simulink model "simulation_upgrade"  (R2024b)
settings: Solver=ode1be  StartTime=0.0  StopTime=10  FixedStep=0.001  RelTol=1e-3
model workspace (MAT data in the model file):
  AMP = 1
  FREQ = 1
  i_abc = 1
values from neighbouring files (symbols this model uses):
  v_WLTP = [0 0 0 0 0 0 0 0 0 0 0 0 ... (180001 elements, 1x180001)]    [v_WLTP.mat]
undefined symbols (not defined in the file or in its folder): A, a_sig, b_sig, C1, C2, C3, Cd, CG_z, downshift, Drive_wheel, Driveshaft, f_blend, f_OVD, fo, front_seat_dist, fs, g, Gearbox, i, i_sig, Inclination, Inertia, Jr2, K, m, M_curve_1, M_curve_2, m_driver, M_N_1, M_N_2, mi_c, mi_s, Mode, N_clutch, n_curve_1, n_curve_2, n_driver, n_max_1, n_max_2, n_shift, n_surfaces, Pl, Planetary, r_eq_clutch, r_geom, r_wheel, rho, Shaft, shift_time, sigma0, sigma1, sigma2, slope_angle, Stage1, Stage2, Stage3, upshift, v0, vel_wind, vs ... (+5)
libraries: simulink x29, slpidlib x3
(part 1 of 9)
settings Model: Creator=menda  LastModifiedBy=menda
settings SolverCC: ZeroCrossAlgorithm=Adaptive
settings DebuggingCC: AlgebraicLoopMsg=none  IgnoredZcDiagnostic=none

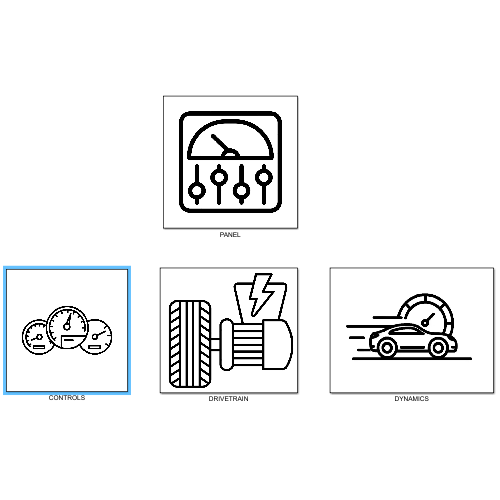
[thumbnail: Simulink's stored preview of the top-level diagram]
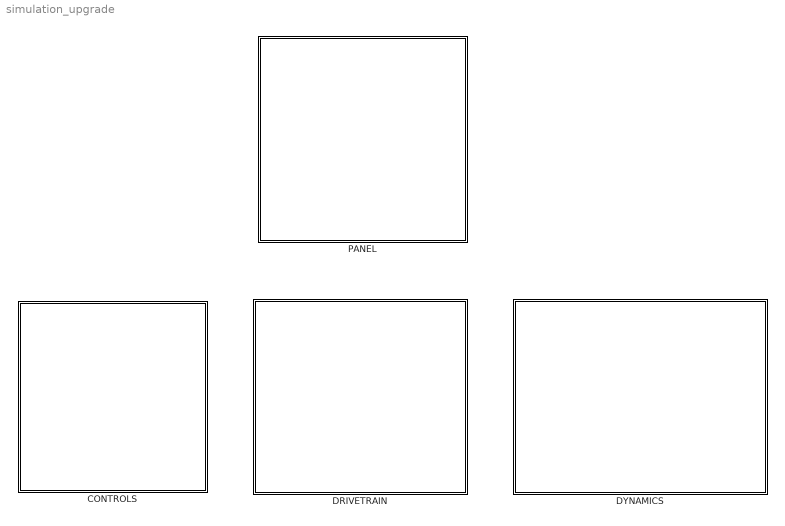
== system simulation_upgrade ==
  CONTROLS : Subsystem
      mask Display: image('images/controls.jpg');
  DRIVETRAIN : Subsystem
      mask Display: image('images/drivetrain_icon.png');
  DYNAMICS : Subsystem
      mask Display: image('images/Dynamics.png');
  PANEL : Subsystem
      mask Display: image('images/panel.jpg');

== system simulation_upgrade/CONTROLS ==
  Main Control Unit : Subsystem  Variant=on
      mask Display: image('images/MCU.jpg');
  Speed Profile : Subsystem
      mask Display: image('images/speedProfile.png');
  Speed control : Subsystem
      mask Display: image('images/speedControl.jpg');
  tag scope: Gear=global, M_MCU=global
  wires:
  Speed Profile/1(V/A) -> Speed control/2(v Target)  "v/a"
  Speed control/1(M) -> Main Control Unit/1(M_Driver)
  [Speed] -> Speed control/1(V fdbk)
  Main Control Unit/1(M_MCU) -> [M_MCU]  "Torque"
  Main Control Unit/2(Gear) -> [Gear]  "Gear"

== system simulation_upgrade/DRIVETRAIN ==
  Engine : Subsystem  Variant=on
      mask Display: image('images/engine.jpg');
  Transmission : Subsystem
      mask Display: image('images/transmission.jpg');
  Wheel Model : Subsystem
      mask Display: image('images/wheel_model.jpg');
  Zero : Constant  Value=0  OutDataTypeStr=Inherit: Inherit via back propagation
  tag scope: F_wheel=global, M_engine=global
  wires:
  Engine/1(M_engine) -> Transmission/1(M_engine), [M_engine]
  Wheel Model/1("  ") -> [F_wheel]  "F_wheels"
  [M_MCU] -> Engine/1(M_MCU)
  Zero/1 -> Wheel Model/3(M_break)
  Transmission/1(M_tra) -> Wheel Model/2(M_tra)
  [V_load] -> Wheel Model/1(Vload)

== system simulation_upgrade/DYNAMICS ==
  Aerodynamic Forces : Subsystem
      mask Display: image('images/aerodynamic.png');
  Inclination : Subsystem
      mask Display: image('images/slope.jpg');
  Load Transfer : Subsystem
      mask Display: image('images/Load_transfer.png');
  Rolling Resistance : Subsystem
      mask Display: image('images/rolling_resistance.png');
  Sum : Sum  Inputs=-+-
  Vehicle Dynamics : Subsystem
      mask Display: image('images/Dynamics.png');
  tag scope: Speed=global, V_load=global
  wires:
  Sum/1 -> Vehicle Dynamics/1(Ft)  "F_tractive"
  Rolling Resistance/1(F) -> Sum/2  "Fx"
  Inclination/1(F_G) -> Sum/3  "F_G"
  Aerodynamic Forces/1(Fa) -> Sum/1  "D_A"
  Vehicle Dynamics/1(v) -> [Speed]  "v"
  [Speed] -> Aerodynamic Forces/1(v_x), Rolling Resistance/1(v_x)
  Load Transfer/1(Fz) -> [V_load]
  Vehicle Dynamics/2(acc) -> Load Transfer/1(acc)
  Inclination/2(theta) -> Load Transfer/2(theta)
  [F_wheel] -> Rolling Resistance/2(Fw)
  [V_load] -> Rolling Resistance/3(Fz)

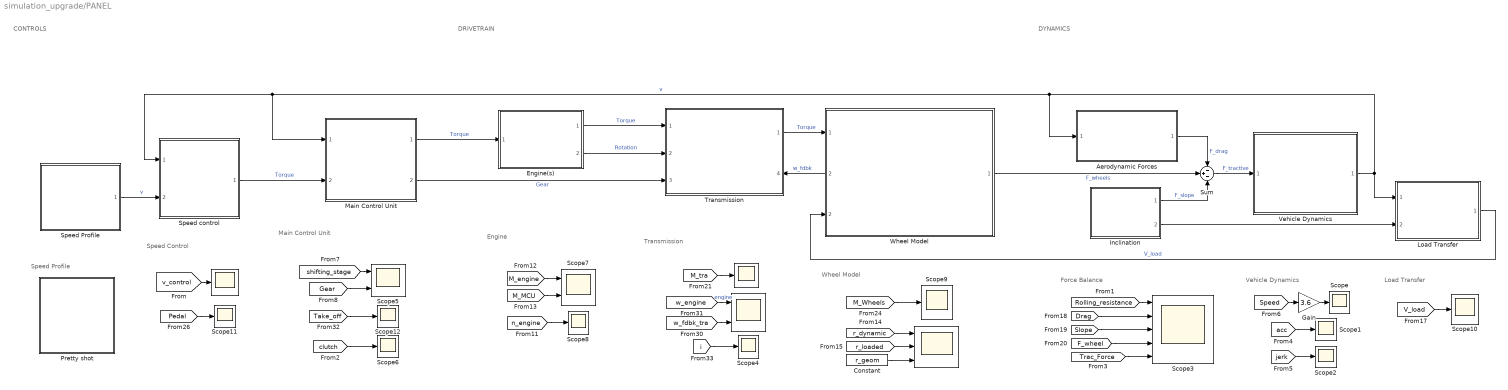
== system simulation_upgrade/PANEL ==
  note: Load Transfer
  note: Vehicle Dynamics
  note: Force Balance
  note: Speed Profile
  note: Transmission
  note: Main Control Unit
  note: Speed Control
  note: DYNAMICS
  note: CONTROLS
  note: DRIVETRAIN
  note: Engine
  note: Wheel Model
  " " : Scope
  "  " : Scope  NumInputPorts=3
  "        " : Scope  NumInputPorts=2
  "                " : Scope
  Aerodynamic Forces : Subsystem
      mask Display: image('images/aerodynamic.png');
  Constant : Constant  Value=r_geom
  Engine(s) : Subsystem
      mask Display: image('images/engine.jpg');
  Gain : Gain  Gain=3.6
  Inclination : Subsystem
      mask Display: image('images/slope.jpg');
  Load Transfer : Subsystem
      mask Display: image('images/Load_transfer.png');
  Main Control Unit : Subsystem
      mask Display: image('images/MCU.jpg');
  Pretty shot : Subsystem
  Scope{,1..2,4,6,8..12} (10 alike) : Scope
  Scope3 : Scope  NumInputPorts=5
  Scope5 : Scope  NumInputPorts=2
  Scope7 : Scope  NumInputPorts=2
  Speed Profile : Subsystem
      mask Display: image('images/speedProfile.png');
  Speed control : Subsystem
      mask Display: image('images/speedControl.jpg');
  Sum : Sum  Inputs=-+-
  Transmission : Subsystem
      settings: PortSchema="{\"entries\":[{\"content\":{\"sides\":[{\"content\":{\"connectorIds\":[\"In1\",\"In2\",\"In3\"]},\"type\":\"ConnectorPlacement.EquallySpacedRectSide\",\"uuid\":\"938dd209-6296-408a-9216-1c78db94ab7e\"},{\"content\":{\"connectorIds\":[\"Out1\",\"In4\"],\"side\":\"RIGHT\"},\"type\":\"ConnectorPlacement.EquallySpacedRectSide\",\"uuid\":\"09e50ecb-d14d-4cb9-a827-f943ac6e708a\"},{\"content\":{\"side\":\"TOP\"},\"type\":\"ConnectorPlacement.EquallySpacedRectSide\",\"uuid\":\"2d9a187e-939f-4518-982a-97ec647a77f4\"}]},\"type\":\"ConnectorPlacement.EquallySpacedConnector\",\"uuid\":\"677d1034-9393-4137-a143-928c8b2a4264\"}],\"packageUris\":[\"http://schema.mathworks.com/mf0/Connector/R2020b\"],\"version\":\"1.0\"}"
      mask Display: image('images/transmission.jpg');
  Vehicle Dynamics : Subsystem
      mask Display: image('images/Dynamics.png');
  Wheel Model : Subsystem
      settings: PortSchema="{\"entries\":[{\"content\":{\"sides\":[{\"content\":{\"connectorIds\":[\"In1\",\"Out2\",\"In2\"]},\"type\":\"ConnectorPlacement.EquallySpacedRectSide\",\"uuid\":\"938dd209-6296-408a-9216-1c78db94ab7e\"},{\"content\":{\"connectorIds\":[\"Out1\"],\"side\":\"RIGHT\"},\"type\":\"ConnectorPlacement.EquallySpacedRectSide\",\"uuid\":\"09e50ecb-d14d-4cb9-a827-f943ac6e708a\"},{\"content\":{\"side\":\"TOP\"},\"type\":\"ConnectorPlacement.EquallySpacedRectSide\",\"uuid\":\"2d9a187e-939f-4518-982a-97ec647a77f4\"}]},\"type\":\"ConnectorPlacement.EquallySpacedConnector\",\"uuid\":\"677d1034-9393-4137-a143-928c8b2a4264\"}],\"packageUris\":[\"http://schema.mathworks.com/mf0/Connector/R2020b\"],\"version\":\"1.0\"}"
      mask Display: image('images/wheel_model.jpg');
  wires:
  [v_control] -> "                "/1
  [Speed] -> Gain/1
  [acc] -> Scope1/1
  [Trac_Force] -> Scope3/5
  [jerk] -> Scope2/1
  [Gear] -> Scope5/2
  [shifting_stage] -> Scope5/1
  [M_engine] -> Scope7/1
  [M_MCU] -> Scope7/2
  [n_engine] -> Scope8/1
  Inclination/1(" ") -> Sum/3  "F_slope"
  Sum/1 -> Vehicle Dynamics/1(" ")  "F_tractive"
  Load Transfer/1("  ") -> Wheel Model/2("  ")  "V_load"
  Speed Profile/1(" ") -> Speed control/2("    ")  "v"
  Main Control Unit/1("    ") -> Engine(s)/1("  ")  "Torque"
  Aerodynamic Forces/1("  ") -> Sum/1  "F_drag"
  Vehicle Dynamics/1("  ") -> Aerodynamic Forces/1(" "), Speed control/1(" "), Main Control Unit/1(" "), Load Transfer/1(" ")  "v"
  Engine(s)/1("             ") -> Transmission/1(" ")  "Torque"
  Wheel Model/1("   ") -> Sum/2  "F_wheels"
  Transmission/1("  ") -> Wheel Model/1(" ")  "Torque"
  Speed control/1("        ") -> Main Control Unit/2("   ")  "Torque"
  Main Control Unit/2("  ") -> Transmission/3("    ")  "Gear"
  [r_dynamic] -> "  "/1
  [r_loaded] -> "  "/2
  Constant/1 -> "  "/3
  [V_load] -> Scope10/1
  [Drag] -> Scope3/2
  [Slope] -> Scope3/3
  [F_wheel] -> Scope3/4
  Inclination/2("   ") -> Load Transfer/2("      ")
  [M_tra] -> " "/1
  [M_Wheels] -> Scope9/1
  [Pedal] -> Scope11/1
  [w_fdbk_tra] -> "        "/2
  Gain/1 -> Scope/1
  [w_engine] -> "        "/1  "engine"
  [Take_off] -> Scope12/1
  [i] -> Scope4/1
  Wheel Model/2("    ") -> Transmission/4("   ")  "w_fdbk"
  Engine(s)/2("              ") -> Transmission/2("     ")  "Rotation"
  [Rolling_resistance] -> Scope3/1
  [clutch] -> Scope6/1

== system simulation_upgrade/CONTROLS/Main Control Unit ==
  note: 1) Add Subsystem or Model blocks as valid variant choices.
      | 2) You cannot connect blocks at this level. At simulation, connectivity is automatically
      | determined, based on the active variant and port name matching.
  M_Driver : Inport
  AMT_MCU : Subsystem  VariantControl=Gearbox == 2
  AT_MCU : Subsystem  VariantControl=Gearbox == 1
  CVT_MCU : Subsystem  VariantControl=Gearbox == 5
  DCT_MCU : Subsystem  VariantControl=Gearbox == 3
  TDT_MCU : Subsystem  VariantControl=Gearbox == 4
  M_MCU : Outport
  Gear : Outport  Port=2

== system simulation_upgrade/CONTROLS/Speed Profile ==
  0% Pedal : Step  Time=0  After=0  SampleTime=0
  AND : Logic  IconShape=distinctive  AllPortsSameDT=off  OutDataTypeStr=boolean
  Add3 : Sum
  Bus Creator : BusCreator  Inputs=2
  Compare To Constant2 : simulink/Logic and Bit Operations/Compare To Constant  relop=>=  const=2  OutDataTypeStr=boolean
  Compare To Constant3 : simulink/Logic and Bit Operations/Compare To Constant  relop=<  const=0.01  OutDataTypeStr=boolean
  Constant : Constant  Value=Mode
  Constant12 : Constant  Value=0.3
  Constant13 : Constant  Value=0
  Constant14 : Constant  Value=0
  Constant15 : Constant  Value=-0.6
  Digital Clock : DigitalClock  SampleTime=0.001
  Digital Clock1 : DigitalClock  SampleTime=0.01
  Gain : Gain  Gain=3.6
  Ramp1 : simulink/Sources/Ramp  slope=1  start=0  InitialOutput=0
  Ramp2 : simulink/Sources/Ramp  slope=-0.5  start=10  InitialOutput=0
  Saturation Dynamic : simulink/Discontinuities/Saturation Dynamic  OutMin=[]  OutMax=[]  OutDataTypeStr=Inherit: Same as second input  OutDataType=fixdt(1, 16)  OutScaling=2^-10  DoSatur=off
  Saturation Dynamic1 : simulink/Discontinuities/Saturation Dynamic  OutMin=[]  OutMax=[]  OutDataTypeStr=Inherit: Same as second input  OutDataType=fixdt(1, 16)  OutScaling=2^-10  DoSatur=off
  Scope25 : Scope
  Scope26 : Scope
  Setpoint Speed (Acceleration) : Step  Time=0  After=80  SampleTime=0
  Setpoint Speed (Acceleration)1 : Step  Time=10  After=-80  SampleTime=0
  Sum : Sum  Inputs=|++
  Switch : Switch  Criteria=u2 > Threshold  Threshold=1  SaturateOnIntegerOverflow=off  InputSameDT=off
  Switch2 : Switch  Criteria=u2 > Threshold  SaturateOnIntegerOverflow=off  InputSameDT=off
  WLTP Profile : Lookup_n-D  NumberOfTableDimensions=1  BreakpointsForDimension1=t  Table=v_WLTP  InternalRulePriority=Speed  RndMeth=Simplest
  V/A : Outport
  wires:
  Setpoint Speed (Acceleration)1/1 -> Sum/2
  Setpoint Speed (Acceleration)/1 -> Sum/1
  Digital Clock/1 -> WLTP Profile/1
  WLTP Profile/1 -> Switch/1
  Constant/1 -> Switch/2
  Sum/1 -> Switch/3
  Switch/1 -> Bus Creator/2  "v_target"
  Constant12/1 -> Saturation Dynamic1/1
  Digital Clock1/1 -> Compare To Constant2/1
  Constant14/1 -> Saturation Dynamic/1
  [Speed] -> Gain/1
  Saturation Dynamic/1 -> Add3/1
  Switch2/1 -> Scope26/1, Bus Creator/1  "pedal"
  Compare To Constant2/1 -> AND/1
  Ramp2/1 -> Saturation Dynamic/2
  AND/1 -> Switch2/2
  Saturation Dynamic1/1 -> Add3/2
  Constant13/1 -> Saturation Dynamic1/3
  Compare To Constant3/1 -> AND/2
  Gain/1 -> Compare To Constant3/1  "v_ist"
  Constant15/1 -> Saturation Dynamic/3
  Add3/1 -> Switch2/3, Scope25/1
  0% Pedal/1 -> Switch2/1  "Pedal Value Limited"
  Ramp1/1 -> Saturation Dynamic1/2
  Bus Creator/1 -> V/A/1

== system simulation_upgrade/CONTROLS/Speed control ==
  V fdbk : Inport
  v Target : Inport  Port=2
  Add : Sum  Inputs=+-
  Bus Creator : BusCreator  Inputs=3
  Bus Selector : BusSelector  OutputSignals=pedal,v_target
  Constant : Constant  Value=Mode
  Constant1 : Constant  Value=Gearbox
  Gain : Gain  Gain=3.6
  Gain1 : Gain  Gain=M_N_1
  Gain2 : Gain  Gain=M_N_2
  Pedal Value Limiter : Saturate  UpperLimit=1  LowerLimit=-1
  Speed Control : slpidlib/PID Controller  Controller=PID  Form=Parallel  TimeDomain=Continuous-time  UseExternalTs=off  SampleTime=-1  IntegratorMethod=Forward Euler  FilterMethod=Forward Euler  ControllerParametersSource=internal  P=0.8  I=0.001  UseKiTs=off  D=0  UseExternalDerivativeSource=off  N=100  UseFilter=on  TunerSelectOption=Transfer Function Based (PID Tuner App)  InitialConditionSource=internal  InitialConditionForIntegrator=0  InitialConditionForFilter=0  DifferentiatorICPrevScaledInput=0  ExternalReset=none  TrackingMode=off  Kt=1  LimitOutput=off  SatLimitsSource=internal  UpperSaturationLimit=inf  LowerSaturationLimit=-inf  LinearizeAsGain=on  AntiWindupMode=none  Kb=1  LimitIntegrator=off  UpperIntegratorSaturationLimit=inf  LowerIntegratorSaturationLimit=-inf  POutMin=[]  POutMax=[]  IOutMin=[]  IOutMax=[]  DOutMin=[]  DOutMax=[]  NOutMin=[]  NOutMax=[]  SumOutMin=[]  SumOutMax=[]  SaturationOutMin=[]  SaturationOutMax=[]  PParamMin=[]  PParamMax=[]  IParamMin=[]  IParamMax=[]  DParamMin=[]  DParamMax=[]  NParamMin=[]  NParamMax=[]  KbParamMin=[]  KbParamMax=[]  KtParamMin=[]  KtParamMax=[]  KbOutMin=[]  KbOutMax=[]  KtOutMin=[]  KtOutMax=[]  IntegratorOutMin=[]  IntegratorOutMax=[]  FilterOutMin=[]  FilterOutMax=[]  SumI1OutMin=[]  SumI1OutMax=[]  SumI2OutMin=[]  SumI2OutMax=[]  SumI3OutMin=[]  SumI3OutMax=[]  SumI4OutMin=[]  SumI4OutMax=[]  SumDOutMin=[]  SumDOutMax=[]  DifferentiatorOutMin=[]  DifferentiatorOutMax=[]  FilterDiffOutCoefMin=[]  FilterDiffOutCoefMax=[]  ReciprocalOutMin=[]  ReciprocalOutMax=[]  SumDenOutMin=[]  SumDenOutMax=[]  SumNumOutMin=[]  SumNumOutMax=[]  DivideOutMin=[]  DivideOutMax=[]  UdiffTsProdOutMin=[]  UdiffTsProdOutMax=[]  NTsProdOutMin=[]  NTsProdOutMax=[]  UintegralTsProdOutMin=[]  UintegralTsProdOutMax=[]  UngainTsProdOutMin=[]  UngainTsProdOutMax=[]  ClampingZeroOutDataTypeStr=Inherit: Inherit via back propagation  ClampingZeroOutMin=[]  ClampingZeroOutMax=[]  FilterDenConstantOutDataTypeStr=Inherit: Inherit via back propagation  FilterDenConstantOutMin=[]  FilterDenConstantOutMax=[]  PCopyOutDataTypeStr=Inherit: Inherit via back propagation  PCopyOutMin=[]  PCopyOutMax=[]  NCopyOutDataTypeStr=Inherit: Inherit via back propagation  NCopyOutMin=[]  NCopyOutMax=[]  IntegratorContinuousStateAttributes=''  IntegratorStateMustResolveToSignalObject=off  IntegratorRTWStateStorageClass=Auto  FilterContinuousStateAttributes=''  FilterStateMustResolveToSignalObject=off  FilterRTWStateStorageClass=Auto  ParallelPVariant=InternalParameters  IdealPVariant=Disabled  IVariant=InternalParameters  DVariant=InternalParameters  IntegratorVariant=Continuous  SatVariant=Disabled  AWVariant=Passthrough  PCopyVariant=Disabled  TRVariant=Disabled  FdbkBlocksVariant=Forward  IdealPFdbkVariant=Disabled  SatFdbkVariant=Disabled  DerivativeFilterVariant=ContFilter  NVariant=InternalParameters  NCopyVariant=Disabled  FilterICVariant=InternalICsFilter  IntegratorICVariant=InternalICs  ExternalResetVariant=Disabled  TRSumVariant=Passthrough  SumFdbkVariant=Disabled  SumVariant=Sum_PID  TsampFilterVariant=InternalTs  TsampNgainVariant=Passthrough  TsampIntegralVariant=Disabled_SignalSpec  ExternalSaturationOutDataTypeStr=Inherit: Same as second input  DerivativeSourceVariant=ErrorSignal  PreIntVariant=InternalPreInt
  Sum : Sum  Inputs=|++
  Switch : Switch  Criteria=u2 > Threshold  Threshold=2  SaturateOnIntegerOverflow=off  InputSameDT=off
  Switch1 : Switch  Criteria=u2 > Threshold  Threshold=3  SaturateOnIntegerOverflow=off  InputSameDT=off
  Transfer Fcn : TransferFcn  Denominator=[0.008 1]
  M : Outport
  tag scope: Pedal=global, v_control=global, v_error=global, v_fdbk=global, v_target=global
  wires:
  Add/1 -> Speed Control/1, [v_error]  "v_error"
  Speed Control/1 -> Pedal Value Limiter/1
  Switch1/1 -> M/1  "Setpoint Torque"
  V fdbk/1 -> Gain/1
  Gain/1 -> [v_fdbk], Add/2  "v_fdbk"
  Transfer Fcn/1 -> Gain1/1, Gain2/1, [Pedal]  "Pedal_value"
  Pedal Value Limiter/1 -> Switch/3
  Constant/1 -> Switch/2
  v Target/1 -> Bus Selector/1
  Bus Selector/1 -> Switch/1  "<pedal>"
  Gain1/1 -> Switch1/3, Sum/2
  Sum/1 -> Switch1/1
  Gain2/1 -> Sum/1
  Constant1/1 -> Switch1/2
  Switch/1 -> Transfer Fcn/1
  [v_target] -> Bus Creator/3  "v_target"
  [v_fdbk] -> Bus Creator/1  "v_fdbk"
  [v_error] -> Bus Creator/2  "v_error"
  Bus Creator/1 -> [v_control]
  Bus Selector/2 -> Add/1, [v_target]  "<v_target>"

== system simulation_upgrade/DRIVETRAIN/Engine ==
  note: 1) Add Subsystem or Model blocks as valid variant choices.
      | 2) You cannot connect blocks at this level. At simulation, connectivity is automatically
      | determined, based on the active variant and port name matching.
  M_MCU : Inport
  AMT_Engine : Subsystem  VariantControl=Gearbox == 2
  AT_Engine : Subsystem  VariantControl=Gearbox == 1
  DCT_Engine : Subsystem  VariantControl=Gearbox == 3
  TDT_Engine : Subsystem  VariantControl=Gearbox == 4
  e-CVT_Engine : Subsystem  VariantControl=Gearbox == 5
  M_engine : Outport

== system simulation_upgrade/DRIVETRAIN/Transmission ==
  M_engine : Inport
  Differential and Driveshafts : Subsystem
      mask Display: image('images/transmission.jpg');
  Gearbox : Subsystem  Variant=on
      mask Display: image('images/branco.png');
  eff_GB : Gain  Gain=0.97
  M_tra : Outport
  wires:
  M_engine/1 -> Gearbox/1(M_engine)
  Gearbox/1(M_Diff) -> eff_GB/1
  eff_GB/1 -> Differential and Driveshafts/1(M_Diff)
  Differential and Driveshafts/1(M_tra) -> M_tra/1

== system simulation_upgrade/DRIVETRAIN/Wheel Model ==
  Vload : Inport
  M_tra : Inport  Port=2
  M_break : Inport  Port=3
  Bus Creator : BusCreator  Inputs=2
  Bus Creator1 : BusCreator  Inputs=2
  Bus Creator2 : BusCreator  Inputs=2
  Bus Selector : BusSelector  OutputSignals=Rear_Vload,Front_Vload
  Constant5 : Constant  Value=Drive_wheel
  Divide2 : Product  Inputs=/*
  Front Wheels : Subsystem
      mask Display: image('images/branco.png');
  Integrator : Integrator
  Multiport Switch : MultiPortSwitch  DataPortOrder=Zero-based contiguous  zeroidx=on  SaturateOnIntegerOverflow=off  InputSameDT=off
  Rear Wheels : Subsystem
      mask Display: image('images/branco.png');
  Sum : Sum  Inputs=+|+
  "  " : Outport
  tag scope: M_Wheels=global, r_dynamic=global, r_loaded=global, w_fdbk_tire=global
  wires:
  Sum/1 -> "  "/1
  Vload/1 -> Bus Selector/1
  Bus Selector/1 -> Rear Wheels/3(Vload)  "<Rear_Vload>"
  Bus Selector/2 -> Front Wheels/1(Vload)  "<Front_Vload>"
  Rear Wheels/1(F_rear_wheels) -> Sum/1  "F_rear"
  Front Wheels/1(F_front_wheels) -> Sum/2  "F_front"
  M_tra/1 -> Rear Wheels/1(M_tra), Front Wheels/2(M_tra)
  M_break/1 -> Front Wheels/3(M_break), Rear Wheels/2(M_break)
  [acc] -> Divide2/2
  Multiport Switch/1 -> Divide2/1
  Integrator/1 -> [w_fdbk_tire]  "w_fdbk_tire"
  Constant5/1 -> Multiport Switch/1
  [r_dyn_rear] -> Bus Creator/2, Multiport Switch/4, Multiport Switch/2
  [r_dyn_front] -> Multiport Switch/3, Bus Creator/1
  Bus Creator/1 -> [r_dynamic]
  Bus Creator1/1 -> [r_loaded]
  [r_loaded_front] -> Bus Creator1/2
  [r_loaded_rear] -> Bus Creator1/1
  Divide2/1 -> Integrator/1
  [M_front_wheels] -> Bus Creator2/1
  [M_rear_wheels] -> Bus Creator2/2
  Bus Creator2/1 -> [M_Wheels]

== system simulation_upgrade/DYNAMICS/Aerodynamic Forces ==
  v_x : Inport
  Add : Sum  Inputs=+-
  Constant : Constant  Value=rho*A*0.5*Cd
  Constant1 : Constant  Value=vel_wind
  Math Function : Math  Operator=square  SignedPower=on
  Product : Product  RndMeth=Zero
  Product2 : Product  RndMeth=Zero
  Sign : Signum
  Fa : Outport  VectorParamsAs1DForOutWhenUnconnected=off
  tag scope: Drag=global
  wires:
  Add/1 -> Math Function/1
  Math Function/1 -> Product/2
  Sign/1 -> Product/1
  Constant/1 -> Product2/2
  Product2/1 -> [Drag], Fa/1  "Drag"
  Constant1/1 -> Add/2
  v_x/1 -> Add/1, Sign/1
  Product/1 -> Product2/1

== system simulation_upgrade/DYNAMICS/Inclination ==
  Constant : Constant  Value=slope_angle
  Constant1 : Constant  Value=Inclination
  Constant8 : Constant  Value=m+n_driver*m_driver
  Constant9 : Constant  Value=g
  Digital Clock : DigitalClock  Commented=on  SampleTime=0.01
  Product : Product  Inputs=3  RndMeth=Zero
  Slope Profile : Lookup_n-D  Commented=on  NumberOfTableDimensions=1  BreakpointsForDimension1=t  Table=i_sig  InternalRulePriority=Speed  RndMeth=Simplest
  Switch : Switch  Criteria=u2 > Threshold  SaturateOnIntegerOverflow=off  InputSameDT=off
  Trigonometric Function : Trigonometry
  F_G : Outport  VectorParamsAs1DForOutWhenUnconnected=off
  theta : Outport  Port=2  VectorParamsAs1DForOutWhenUnconnected=off
  tag scope: Slope=global
  wires:
  Product/1 -> F_G/1, [Slope]  "Slope"
  Constant9/1 -> Product/3
  Switch/1 -> theta/1, Trigonometric Function/1
  Trigonometric Function/1 -> Product/1
  Constant8/1 -> Product/2
  Constant/1 -> Switch/3
  Constant1/1 -> Switch/2
  Digital Clock/1 -> Slope Profile/1
  Slope Profile/1 -> Switch/1

== system simulation_upgrade/DYNAMICS/Load Transfer ==
  acc : Inport
  theta : Inport  Port=2
  Bus Creator : BusCreator  Inputs=2
  Constant : Constant  Value=g*WB_rear_dist
  Constant1 : Constant  Value=n_driver*m_driver*g*front_seat_dist
  Constant2 : Constant  Value=g*(1-WB_rear_dist)
  Constant3 : Constant  Value=n_driver*m_driver*g*(1-front_seat_dist)
  Cos : Trigonometry  Operator=cos
  Delay3 : Delay  DelayLength=1  InputProcessing=Columns as channels (frame based)
  Gain1 : Gain  Gain=CG_z/WB
  Product{,1..5} (6 alike) : Product
  Sum : Sum  Inputs=|++
  Sum1 : Sum  Inputs=-+|
  Sum2 : Sum  Inputs=++|
  Sum3 : Sum  Inputs=++|
  Fz : Outport
  tag scope: Vload_front=global, Vload_rear=global
  wires:
  Sum/1 -> Product/1
  Gain1/1 -> Sum/2, Sum1/1
  Sum1/1 -> Product1/2
  Sum3/1 -> Bus Creator/2, [Vload_front]  "Front_Vload"
  Sum2/1 -> Bus Creator/1, [Vload_rear]  "Rear_Vload"
  [m_eff] -> Product/2, Product1/1
  Constant/1 -> Product2/2
  Constant2/1 -> Product3/1
  Bus Creator/1 -> Fz/1
  acc/1 -> Delay3/1
  Delay3/1 -> Gain1/1
  Product/1 -> Sum2/1
  Product1/1 -> Sum3/1
  Constant1/1 -> Product4/1
  Constant3/1 -> Product5/2
  Product2/1 -> Sum/1
  Product3/1 -> Sum1/2
  theta/1 -> Cos/1
  Cos/1 -> Product4/2, Product2/1, Product3/2, Product5/1
  Product4/1 -> Sum2/2
  Product5/1 -> Sum3/2

== system simulation_upgrade/DYNAMICS/Rolling Resistance ==
  v_x : Inport
  Fw : Inport  Port=2
  Fz : Inport  Port=3
  Abs : Abs  SaturateOnIntegerOverflow=off
  Abs2 : Abs  SaturateOnIntegerOverflow=off
  Bus Selector : BusSelector  OutputSignals=Rear_Vload,Front_Vload
  Constant : Constant  Value=2.5
  Constant1 : Constant  Value=fo
  Delay : Delay  DelayLength=1  InputProcessing=Columns as channels (frame based)
  Gain : Gain  Gain=1/44.7
  Gain1 : Gain  Gain=3.24*fs
  Gain2 : Gain  Gain=-1
  Power : Math  Operator=pow
  Product : Product
  Saturation Dynamic : simulink/Discontinuities/Saturation Dynamic  OutMin=[]  OutMax=[]  OutDataTypeStr=Inherit: Same as second input  OutDataType=fixdt(1, 16)  OutScaling=2^-10  DoSatur=off
  Scope : Scope
  Step : Step  Time=0  After=0  SampleTime=0
  Sum : Sum  Inputs=|++
  Sum1 : Sum  Inputs=+-|
  Sum2 : Sum  Inputs=+|+
  Switch : Switch  SaturateOnIntegerOverflow=off  InputSameDT=off
  F : Outport
  tag scope: Rolling_resistance=global
  wires:
  Gain/1 -> Power/1
  Constant/1 -> Power/2
  Power/1 -> Gain1/1
  Gain1/1 -> Sum/1
  Constant1/1 -> Sum/2
  Sum/1 -> Scope/1, Product/2  "f_roll"
  Fz/1 -> Bus Selector/1
  Product/1 -> Switch/1
  Saturation Dynamic/1 -> Sum1/2, [Rolling_resistance]  "rolling_resistance"
  Fw/1 -> Sum1/1, Abs/1
  v_x/1 -> Delay/1
  Abs2/1 -> Switch/2
  Sum1/1 -> F/1
  Bus Selector/1 -> Sum2/1  "<Rear_Vload>"
  Sum2/1 -> Product/1
  Bus Selector/2 -> Sum2/2  "<Front_Vload>"
  Delay/1 -> Gain/1, Abs2/1
  Switch/1 -> Saturation Dynamic/2
  Gain2/1 -> Saturation Dynamic/3
  Step/1 -> Switch/3
  Abs/1 -> Gain2/1, Saturation Dynamic/1

== system simulation_upgrade/DYNAMICS/Vehicle Dynamics ==
  Ft : Inport
  Constant2 : Constant  Value=v0
  Derivative : Derivative
  Divide : Product  Inputs=*/
  Effective mass : Subsystem
  Integrator1 : Integrator  InitialConditionSource=external
  Saturation : Saturate  UpperLimit=3*m*g/2  LowerLimit=-3*m*g/2
  Scope : Scope  NumInputPorts=3
  Speed Saturation1 : Saturate  UpperLimit=2*pi*r_geom*n_max_1/(60*i.min)  LowerLimit=0
  v : Outport
  acc : Outport  Port=2
  tag scope: Trac_Force=global, acc=global, jerk=global
  wires:
  Ft/1 -> Saturation/1, Scope/1, [Trac_Force]  "F_tractive"
  Integrator1/1 -> Speed Saturation1/1  "v_x"
  Derivative/1 -> [jerk]
  Effective mass/1(m_eff) -> Divide/2
  Saturation/1 -> Divide/1, Scope/2
  Divide/1 -> Integrator1/1, Derivative/1, acc/1, Scope/3, [acc]  "acc"
  Constant2/1 -> Integrator1/2
  Speed Saturation1/1 -> v/1

== system simulation_upgrade/PANEL/Aerodynamic Forces ==
  " " : Inport
  "  " : Outport
  wires:
  " "/1 -> "  "/1

== system simulation_upgrade/PANEL/Engine(s) ==
  "  " : Inport
  "             " : Outport
  "              " : Outport  Port=2
  wires:
  "  "/1 -> "             "/1

== system simulation_upgrade/PANEL/Inclination ==
  Constant : Constant
  " " : Outport
  "   " : Outport  Port=2
  wires:
  Constant/1 -> "   "/1, " "/1

== system simulation_upgrade/PANEL/Load Transfer ==
  " " : Inport
  "      " : Inport  Port=2
  Terminator : Terminator
  "  " : Outport
  wires:
  " "/1 -> "  "/1
  "      "/1 -> Terminator/1

== system simulation_upgrade/PANEL/Main Control Unit ==
  " " : Inport
  "   " : Inport  Port=2
  Chart : Stateflow chart  Commented=on  TreatAsAtomicUnit=on
  "    " : Outport
  "  " : Outport  Port=2
  wires:
  " "/1 -> Chart/1(" ")
  "   "/1 -> Chart/2("   ")
  Chart/2("    ") -> "    "/1
  Chart/1("  ") -> "  "/1

== system simulation_upgrade/PANEL/Pretty shot ==
  "Aerodynamic Forces " : Subsystem
      mask Display: image('images/aerodynamic.png');
  "Engine(s) " : Subsystem
      settings: PortSchema="{\"entries\":[{\"content\":{\"sides\":[{\"content\":{},\"type\":\"ConnectorPlacement.EquallySpacedRectSide\",\"uuid\":\"ac5fb7f4-8dc2-4c60-98c0-b32a7c0962c0\"},{\"content\":{\"connectorIds\":[\"Out1\",\"Out2\"],\"side\":\"RIGHT\"},\"type\":\"ConnectorPlacement.EquallySpacedRectSide\",\"uuid\":\"b7133a62-cb88-4836-b384-7b1ee67f5a46\"},{\"content\":{\"connectorIds\":[\"In1\"],\"side\":\"TOP\"},\"type\":\"ConnectorPlacement.EquallySpacedRectSide\",\"uuid\":\"f8e13883-115b-42d7-970b-6e45a84dda6f\"},{\"content\":{\"side\":\"BOTTOM\"},\"type\":\"ConnectorPlacement.EquallySpacedRectSide\",\"uuid\":\"500f1a98-e247-4b4c-a18f-57d00a98d574\"}]},\"type\":\"ConnectorPlacement.EquallySpacedConnector\",\"uuid\":\"d392102a-fa12-401e-96eb-94eaccf256c5\"}],\"packageUris\":[\"http://schema.mathworks.com/mf0/Connector/R2020b\"],\"version\":\"1.0\"}"
      mask Display: image('images/engine2.jpg');
  "Inclination " : Subsystem
      mask Display: image('images/slope.jpg');
  "Load Transfer " : Subsystem
      settings: PortSchema="{\"entries\":[{\"content\":{\"sides\":[{\"content\":{\"connectorIds\":[\"In1\"]},\"type\":\"ConnectorPlacement.EquallySpacedRectSide\",\"uuid\":\"26581e23-f4af-4a6b-94dc-24984d7cf9dd\"},{\"content\":{\"connectorIds\":[\"Out1\",\"In2\"],\"side\":\"RIGHT\"},\"type\":\"ConnectorPlacement.EquallySpacedRectSide\",\"uuid\":\"dc974c34-bd2c-4374-a001-b5c53f67a3d1\"},{\"content\":{\"side\":\"TOP\"},\"type\":\"ConnectorPlacement.EquallySpacedRectSide\",\"uuid\":\"199156e0-9732-4241-ab5b-4e4dfddfabae\"}]},\"type\":\"ConnectorPlacement.EquallySpacedConnector\",\"uuid\":\"d2a32550-3940-404c-bc97-4724ab74b5d6\"}],\"packageUris\":[\"http://schema.mathworks.com/mf0/Connector/R2020b\"],\"version\":\"1.0\"}"
      mask Display: image('images/Load_transfer.png');
  "Main Control Unit " : Subsystem
      settings: PortSchema="{\"entries\":[{\"content\":{\"sides\":[{\"content\":{\"connectorIds\":[\"In1\",\"In2\"]},\"type\":\"ConnectorPlacement.EquallySpacedRectSide\",\"uuid\":\"b8fd4e6d-8e53-4c18-9f6d-747eb079d798\"},{\"content\":{\"connectorIds\":[\"Out1\"],\"side\":\"RIGHT\"},\"type\":\"ConnectorPlacement.EquallySpacedRectSide\",\"uuid\":\"2557e908-cd18-4a3e-b3a6-cb286cbd4d67\"},{\"content\":{\"side\":\"TOP\"},\"type\":\"ConnectorPlacement.EquallySpacedRectSide\",\"uuid\":\"b9022aa8-32dd-4520-9d7b-0035f068fa03\"},{\"content\":{\"connectorIds\":[\"Out2\"],\"side\":\"BOTTOM\"},\"type\":\"ConnectorPlacement.EquallySpacedRectSide\",\"uuid\":\"03495357-ab9a-4889-8bdc-80670051615f\"}]},\"type\":\"ConnectorPlacement.EquallySpacedConnector\",\"uuid\":\"266d5008-05ee-4fe5-82db-1148b4f01b90\"}],\"packageUris\":[\"http://schema.mathworks.com/mf0/Connector/R2020b\"],\"version\":\"1.0\"}"
      mask Display: image('images/MCU.jpg');
  "Speed Profile " : Subsystem
      settings: PortSchema="{\"entries\":[{\"content\":{\"sides\":[{\"content\":{},\"type\":\"ConnectorPlacement.EquallySpacedRectSide\",\"uuid\":\"ecf4b2d3-f448-439a-be96-5b35a4fd23fb\"},{\"content\":{\"side\":\"RIGHT\"},\"type\":\"ConnectorPlacement.EquallySpacedRectSide\",\"uuid\":\"9f661ef6-dada-4229-be93-12e76a82dfa4\"},{\"content\":{\"side\":\"TOP\"},\"type\":\"ConnectorPlacement.EquallySpacedRectSide\",\"uuid\":\"ac4e96df-6f30-4a9f-b005-38b2f14b4e0b\"},{\"content\":{\"connectorIds\":[\"Out1\"],\"side\":\"BOTTOM\"},\"type\":\"ConnectorPlacement.EquallySpacedRectSide\",\"uuid\":\"91599a8c-5439-4e2c-bf63-97578b375873\"}]},\"type\":\"ConnectorPlacement.EquallySpacedConnector\",\"uuid\":\"37a2ef72-73af-4705-a390-0aab74e23ce3\"}],\"packageUris\":[\"http://schema.mathworks.com/mf0/Connector/R2020b\"],\"version\":\"1.0\"}"
      mask Display: image('images/speedProfile.png');
  "Speed control " : Subsystem
      settings: PortSchema="{\"entries\":[{\"content\":{\"sides\":[{\"content\":{\"connectorIds\":[\"In1\"]},\"type\":\"ConnectorPlacement.EquallySpacedRectSide\",\"uuid\":\"f4f8b741-b6a2-4dd4-8da5-7f5af22d781d\"},{\"content\":{\"connectorIds\":[\"Out1\",\"Out2\"],\"side\":\"RIGHT\"},\"type\":\"ConnectorPlacement.EquallySpacedRectSide\",\"uuid\":\"587018a4-7c30-4665-afa4-c8ee6c136d05\"},{\"content\":{\"side\":\"TOP\"},\"type\":\"ConnectorPlacement.EquallySpacedRectSide\",\"uuid\":\"e2f3ce37-0f8f-4868-8f23-b8af4c8da06c\"},{\"content\":{\"connectorIds\":[\"In2\"],\"side\":\"BOTTOM\"},\"type\":\"ConnectorPlacement.EquallySpacedRectSide\",\"uuid\":\"1d00021e-93f8-4c87-820c-5d1d8ace6fcf\"}]},\"type\":\"ConnectorPlacement.EquallySpacedConnector\",\"uuid\":\"75917b60-5051-4813-9ca4-a890de563abe\"}],\"packageUris\":[\"http://schema.mathworks.com/mf0/Connector/R2020b\"],\"version\":\"1.0\"}"
      mask Display: image('images/speedControl.jpg');
  Sum1 : Sum  Inputs=-+-
  "Transmission " : Subsystem
      settings: PortSchema="{\"entries\":[{\"content\":{\"sides\":[{\"content\":{\"connectorIds\":[\"In1\",\"In2\"]},\"type\":\"ConnectorPlacement.EquallySpacedRectSide\",\"uuid\":\"938dd209-6296-408a-9216-1c78db94ab7e\"},{\"content\":{\"connectorIds\":[\"Out1\",\"In4\"],\"side\":\"RIGHT\"},\"type\":\"ConnectorPlacement.EquallySpacedRectSide\",\"uuid\":\"09e50ecb-d14d-4cb9-a827-f943ac6e708a\"},{\"content\":{\"connectorIds\":[\"In3\"],\"side\":\"TOP\"},\"type\":\"ConnectorPlacement.EquallySpacedRectSide\",\"uuid\":\"2d9a187e-939f-4518-982a-97ec647a77f4\"},{\"content\":{\"side\":\"BOTTOM\"},\"type\":\"ConnectorPlacement.EquallySpacedRectSide\",\"uuid\":\"e0bb1154-cc7a-419b-854d-2f1522bbb79c\"}]},\"type\":\"ConnectorPlacement.EquallySpacedConnector\",\"uuid\":\"677d1034-9393-4137-a143-928c8b2a4264\"}],\"packageUris\":[\"http://schema.mathworks.com/mf0/Connector/R2020b\"],\"version\":\"1.0\"}"
      mask Display: image('images/transmission.jpg');
  "Vehicle Dynamics " : Subsystem
      mask Display: image('images/Dynamics.png');
  "Wheel Model " : Subsystem
      settings: PortSchema="{\"entries\":[{\"content\":{\"sides\":[{\"content\":{\"connectorIds\":[\"In1\",\"In2\",\"Out2\"]},\"type\":\"ConnectorPlacement.EquallySpacedRectSide\",\"uuid\":\"938dd209-6296-408a-9216-1c78db94ab7e\"},{\"content\":{\"connectorIds\":[\"Out1\"],\"side\":\"RIGHT\"},\"type\":\"ConnectorPlacement.EquallySpacedRectSide\",\"uuid\":\"09e50ecb-d14d-4cb9-a827-f943ac6e708a\"},{\"content\":{\"side\":\"TOP\"},\"type\":\"ConnectorPlacement.EquallySpacedRectSide\",\"uuid\":\"2d9a187e-939f-4518-982a-97ec647a77f4\"}]},\"type\":\"ConnectorPlacement.EquallySpacedConnector\",\"uuid\":\"677d1034-9393-4137-a143-928c8b2a4264\"}],\"packageUris\":[\"http://schema.mathworks.com/mf0/Connector/R2020b\"],\"version\":\"1.0\"}"
      mask Display: image('images/wheel_model.jpg');
  wires:
  "Main Control Unit "/1("  ") -> "Transmission "/3("    ")  "Gear"
  "Vehicle Dynamics "/1("  ") -> "Speed control "/2(" "), "Aerodynamic Forces "/1(" "), "Load Transfer "/1(" ")  "v_fdbk"
  "Transmission "/1("  ") -> "Wheel Model "/2(" ")  "Torque"
  "Load Transfer "/1("  ") -> "Wheel Model "/1("  ")  "F_z"
  "Speed Profile "/1(" ") -> "Speed control "/1("    ")  "v_in"
  "Wheel Model "/1("   ") -> Sum1/2  "F_x"
  "Speed control "/2("        ") -> "Main Control Unit "/2("   ")  "Torque"
  "Engine(s) "/2("              ") -> "Transmission "/2("     ")  "w"
  "Engine(s) "/1("             ") -> "Transmission "/1(" ")  "Torque"
  "Speed control "/1("         ") -> "Main Control Unit "/1(" ")  "Pedal"
  "Inclination "/1("   ") -> "Load Transfer "/2("      ")  "theta"
  "Wheel Model "/2("    ") -> "Transmission "/4("   ")  "w_fdbk"
  "Inclination "/2(" ") -> Sum1/1  "F_G"
  "Aerodynamic Forces "/1("  ") -> Sum1/3  "D_A"
  "Main Control Unit "/2("    ") -> "Engine(s) "/1("  ")  "Torque"
  Sum1/1 -> "Vehicle Dynamics "/1(" ")

== system simulation_upgrade/PANEL/Speed Profile ==
  Constant : Constant
  " " : Outport
  wires:
  Constant/1 -> " "/1

== system simulation_upgrade/PANEL/Speed control ==
  " " : Inport
  "    " : Inport  Port=2
  Terminator : Terminator
  "        " : Outport
  wires:
  "    "/1 -> "        "/1
  " "/1 -> Terminator/1

== system simulation_upgrade/PANEL/Transmission ==
  " " : Inport
  "     " : Inport  Port=2
  "    " : Inport  Port=3
  "   " : Inport  Port=4
  "  " : Outport
  wires:
  " "/1 -> "  "/1

== system simulation_upgrade/PANEL/Vehicle Dynamics ==
  " " : Inport
  "  " : Outport
  wires:
  " "/1 -> "  "/1

== system simulation_upgrade/PANEL/Wheel Model ==
  " " : Inport
  "  " : Inport  Port=2
  "   " : Outport
  "    " : Outport  Port=2
  wires:
  " "/1 -> "   "/1
  "  "/1 -> "    "/1
